simulink model "PMI"  (R2021a)
settings: Solver=VariableStepAuto  StartTime=0.0  StopTime=20  RelTol=1e-3
undefined symbols (not defined in the file or in its folder): i
settings Model: Creator=Santiago  LastModifiedBy=Santiago

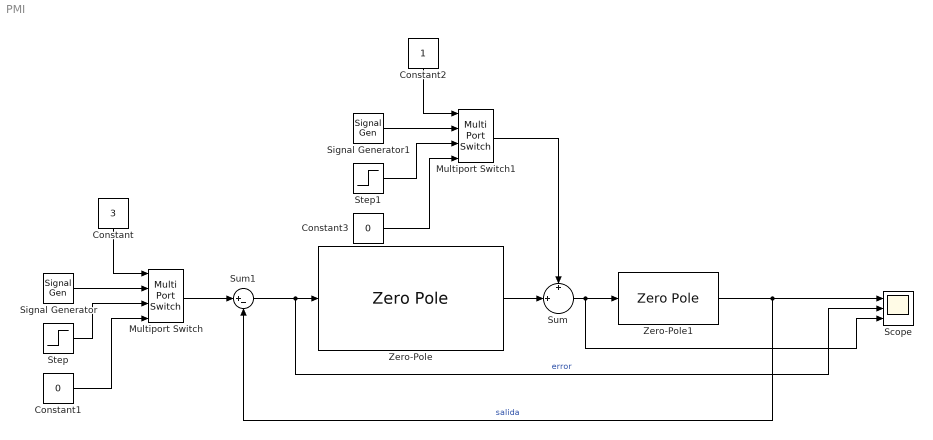
== system PMI ==
  Constant : Constant  Value=3
  Constant1 : Constant  Value=0
  Constant2 : Constant
  Constant3 : Constant  Value=0
  Multiport Switch : MultiPortSwitch
  Multiport Switch1 : MultiPortSwitch
  Scope : Scope  NumInputPorts=3
  Signal Generator : SignalGenerator  Units=rad/sec
  Signal Generator1 : SignalGenerator  Units=rad/sec
  Step : Step  SampleTime=0
  Step1 : Step  SampleTime=0
  Sum : Sum  Inputs=+|+||
  Sum1 : Sum  Inputs=|+-
  Zero-Pole : ZeroPole  Zeros=[-1 -1 -1 -1 -1]  Poles=[i -i -100 -100 -100]
  Zero-Pole1 : ZeroPole  Zeros=[]  Poles=[1 -1 0]
  wires:
  Constant1/1 -> Multiport Switch/4
  Constant/1 -> Multiport Switch/1
  Signal Generator/1 -> Multiport Switch/2
  Step/1 -> Multiport Switch/3
  Multiport Switch/1 -> Sum1/1
  Constant3/1 -> Multiport Switch1/4
  Constant2/1 -> Multiport Switch1/1
  Signal Generator1/1 -> Multiport Switch1/2
  Step1/1 -> Multiport Switch1/3
  Multiport Switch1/1 -> Sum/1
  Zero-Pole/1 -> Sum/2
  Sum1/1 -> Scope/2, Zero-Pole/1  "error"
  Sum/1 -> Scope/3, Zero-Pole1/1
  Zero-Pole1/1 -> Sum1/2, Scope/1  "salida"
